simulink library "calcFluidDynamicLoads"  (R2020a)
settings: Solver=VariableStepAuto  StartTime=0.0  StopTime=10.0  RelTol=1e-3
undefined symbols (not defined in the file): fluidDensity, fluidMomentArms, fluidRefArea, vcl, wingTips
libraries: vrlib x3, clAndCdCalculator_cl x1, dynamicPressure_ul x1, alphaBetaLE_ul x1, localApparentWind_ul x1, rotateAboutVec x1
settings Model: Creator=Ayaz  LastModifiedBy=John Jr

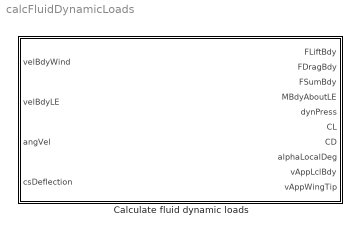
== system calcFluidDynamicLoads ==
  Calculate fluid dynamic loads : Subsystem  mask{aSurf=vcl.portWing, sRef=fluidRefArea, rArm_LE=fluidMomentArms(:,1), rTip_LE=wingTips(:,1), fluidDensity=fluidDensity}
      mask prompts: aSurf "Aerosurf object"; sRef "Reference area"; rArm_LE "Moment arm wrt wing LE"; rTip_LE "Surface tip wrt wing LE"; fluidDensity "Fluid density"

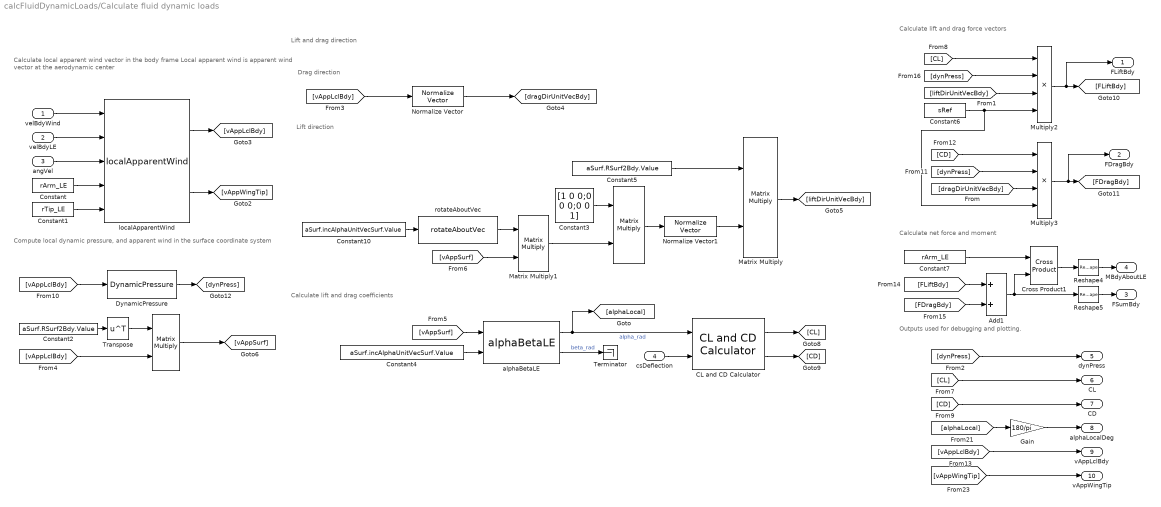
== system calcFluidDynamicLoads/Calculate fluid dynamic loads ==
  note: Lift and drag direction
  note: Lift direction
  note: Drag direction
  note: Compute local dynamic pressure,
      | and apparent wind in the surface coordinate system
  note: Calculate local apparent wind vector in the body frame
      | Local apparent wind is apparent wind vector at the aerodynamic center
  note: Calculate lift and drag coefficients
  note: Calculate net force and moment
  note: Outputs used for debugging and plotting.
  note: Calculate lift and drag force vectors
  velBdyWind : Inport
  velBdyLE : Inport  Port=2
  angVel : Inport  Port=3
  csDeflection : Inport  Port=4
  " " : Product  Multiplication=Matrix(*)
  "  " : Product  Multiplication=Matrix(*)
  Add1 : Sum
  CL and CD Calculator : clAndCdCalculator_cl/CL and CD Calculator  aSurf=0
  Constant : Constant  Value=rArm_LE  VectorParams1D=off
  Constant1 : Constant  Value=rTip_LE  VectorParams1D=off
  Constant10 : Constant  Value=aSurf.incAlphaUnitVecSurf.Value  VectorParams1D=off
  Constant2 : Constant  Value=aSurf.RSurf2Bdy.Value  VectorParams1D=off
  Constant3 : Constant  Value=[1 0 0;0 0 0;0 0 1]  VectorParams1D=off
  Constant4 : Constant  Value=aSurf.incAlphaUnitVecSurf.Value  VectorParams1D=off
  Constant5 : Constant  Value=aSurf.RSurf2Bdy.Value  VectorParams1D=off
  Constant6 : Constant  Value=sRef
  Constant7 : Constant  Value=rArm_LE  VectorParams1D=off
  Cross Product1 : vrlib/Utilities/Cross Product
  DynamicPressure : dynamicPressure_ul/DynamicPressure  rho=fluidDensity
  Gain : Gain  Gain=180/pi
  Matrix Multiply : Product  Multiplication=Matrix(*)
  Matrix Multiply1 : Product  Multiplication=Matrix(*)
  Multiply2 : Product  Inputs=4
  Multiply3 : Product  Inputs=4
  Normalize Vector : vrlib/Utilities/Normalize Vector  maxzero=0
  Normalize Vector1 : vrlib/Utilities/Normalize Vector  maxzero=0
  Reshape4 : Reshape  OutputDimensionality=Column vector (2-D)
  Reshape5 : Reshape  OutputDimensionality=Column vector (2-D)
  Terminator : Terminator
  Transpose : Math  Operator=transpose  SignedPower=on  SaturateOnIntegerOverflow=on
  alphaBetaLE : alphaBetaLE_ul/alphaBetaLE  SystemSampleTime=-1  Latency=0  AutoFrameSizeCalculation=off
  localApparentWind : localApparentWind_ul/localApparentWind  SystemSampleTime=-1  Latency=0  AutoFrameSizeCalculation=off
  rotateAboutVec : rotateAboutVec/rotateAboutVec  ang=90
  FLiftBdy : Outport  VectorParamsAs1DForOutWhenUnconnected=off
  FDragBdy : Outport  Port=2  VectorParamsAs1DForOutWhenUnconnected=off
  FSumBdy : Outport  Port=3  VectorParamsAs1DForOutWhenUnconnected=off
  MBdyAboutLE : Outport  Port=4  PortDimensions=[3 1]  VectorParamsAs1DForOutWhenUnconnected=off
  dynPress : Outport  Port=5  VectorParamsAs1DForOutWhenUnconnected=off
  CL : Outport  Port=6  VectorParamsAs1DForOutWhenUnconnected=off
  CD : Outport  Port=7  VectorParamsAs1DForOutWhenUnconnected=off
  alphaLocalDeg : Outport  Port=8  VectorParamsAs1DForOutWhenUnconnected=off
  vAppLclBdy : Outport  Port=9  VectorParamsAs1DForOutWhenUnconnected=off
  vAppWingTip : Outport  Port=10  VectorParamsAs1DForOutWhenUnconnected=off
  wires:
  velBdyWind/1 -> localApparentWind/1
  velBdyLE/1 -> localApparentWind/2
  angVel/1 -> localApparentWind/3
  Constant/1 -> localApparentWind/4
  Constant1/1 -> localApparentWind/5
  localApparentWind/1 -> [vAppLclBdy]
  localApparentWind/2 -> [vAppWingTip]
  [vAppLclBdy] -> DynamicPressure/1
  "  "/1 -> [vAppSurf]
  Constant2/1 -> Transpose/1
  [vAppLclBdy] -> "  "/2
  DynamicPressure/1 -> [dynPress]
  Transpose/1 -> "  "/1
  Constant3/1 -> " "/1
  rotateAboutVec/1 -> Matrix Multiply1/1
  Matrix Multiply/1 -> [liftDirUnitVecBdy]
  Normalize Vector1/1 -> Matrix Multiply/2
  Constant10/1 -> rotateAboutVec/1
  Matrix Multiply1/1 -> " "/2
  " "/1 -> Normalize Vector1/1
  Constant5/1 -> Matrix Multiply/1
  [vAppSurf] -> Matrix Multiply1/2
  Normalize Vector/1 -> [dragDirUnitVecBdy]
  [vAppLclBdy] -> Normalize Vector/1
  alphaBetaLE/1 -> [alphaLocal], CL and CD Calculator/1  "alpha_rad"
  Constant4/1 -> alphaBetaLE/2
  CL and CD Calculator/2 -> [CD]
  alphaBetaLE/2 -> Terminator/1  "beta_rad"
  csDeflection/1 -> CL and CD Calculator/2
  [vAppSurf] -> alphaBetaLE/1
  CL and CD Calculator/1 -> [CL]
  Constant6/1 -> Multiply2/4, Multiply3/4
  [vAppLclBdy] -> vAppLclBdy/1
  [dynPress] -> dynPress/1
  [FLiftBdy] -> Add1/1
  [vAppWingTip] -> vAppWingTip/1
  Multiply3/1 -> [FDragBdy], FDragBdy/1
  [dragDirUnitVecBdy] -> Multiply3/3
  [CD] -> CD/1
  [dynPress] -> Multiply2/2
  [alphaLocal] -> Gain/1
  [dynPress] -> Multiply3/2
  [CL] -> CL/1
  [CL] -> Multiply2/1
  [liftDirUnitVecBdy] -> Multiply2/3
  Multiply2/1 -> [FLiftBdy], FLiftBdy/1
  [CD] -> Multiply3/1
  [FDragBdy] -> Add1/2
  Reshape5/1 -> FSumBdy/1
  Cross Product1/1 -> Reshape4/1
  Add1/1 -> Cross Product1/2, Reshape5/1
  Constant7/1 -> Cross Product1/1
  Gain/1 -> alphaLocalDeg/1
  Reshape4/1 -> MBdyAboutLE/1
